simulink model "pi_8_8PSK_sim"  (Simulink 8.3)
settings: Solver=ode45  StartTime=0.0  StopTime=10  MaxStep=1e-3  RelTol=1e-3
libraries: dspobslib x2, commdigbbndpm3 x2, commchan3 x1, commsink2 x1, commutil2 x1, commrandsrc2 x1
settings Model: Creator=hlzhang  LastModifiedBy=hlzhang
settings DataIOCC: SignalLoggingName=sigsOut
settings DebuggingCC: SaveWithParameterizedLinksMsg=none  SignalResolutionControl=TryResolveAllWithWarning  SolverPrmCheckMsg=none  MultiTaskDSMMsg=warning  MultiTaskCondExecSysMsg=none  StateNameClashWarn=none
settings HardwareCC: TargetUnknown=on
settings RTWCC: IncludeERTFirstTime=on

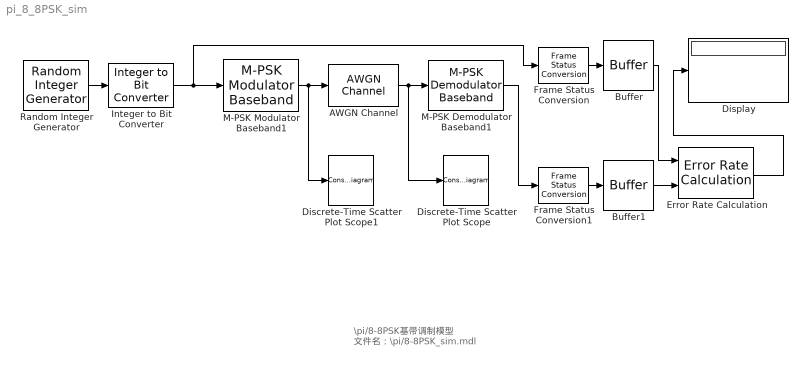
== system pi_8_8PSK_sim ==
  note: \pi/8-8PSK基带调制模型
      | 文件名：\pi/8-8PSK_sim.mdl
  AWGN Channel : commchan3/AWGN Channel  InputProcessing=Inherited (this choice will be removed - see release notes)  seed=67  noiseMode=Variance from mask  EbNodB=10  EsNodB=10  SNRdB=10  bitsPerSym=1  Ps=1  Tsym=1e-3  variance=0.02
  Buffer : Buffer  N=1
  Buffer1 : Buffer  N=1
  Discrete-Time Scatter Plot Scope : ConstellationDiagram  Tag=ScatterPlot  ScopeSpecification=DataTag1
  Discrete-Time Scatter Plot Scope1 : ConstellationDiagram  Tag=ScatterPlot  ScopeSpecification=DataTag2
  Display : Display
  Error Rate Calculation : commsink2/Error Rate Calculation  N=0  st_delay=0  cp_mode=Entire frame  subframe=[]  PMode=Port  WsName=ErrorVec  RsMode2=off  stop=off  numErr=100  maxBits=1e6
  Frame Status Conversion : dspobslib/Frame Status Conversion  growRefPort=off  outframe=Frame-based
  Frame Status Conversion1 : dspobslib/Frame Status Conversion  growRefPort=off  outframe=Frame-based
  Integer to Bit Converter : commutil2/Integer to Bit Converter  nbits=3  signedInputValues=Unsigned  bitOrder=MSB first  outDtype=Inherit via internal rule
  M-PSK Demodulator Baseband1 : commdigbbndpm3/M-PSK Demodulator Baseband  M=8  Ph=pi/8  Dec=Gray  Mapping=[0:7]  OutType=Bit  DecType=Hard decision  VarSource=Dialog  Variance=1  outDtype1=Inherit via internal rule  outDtype2=Inherit via internal rule  derotateFactorWordLen=16
  M-PSK Modulator Baseband1 : commdigbbndpm3/M-PSK Modulator Baseband  M=8  InType=Bit  Enc=Gray  Mapping=[0:7]  Ph=pi/8  outDtype=double  outWordLen=16  outUDDataType=sfix(16)  outFracLenMode=Best precision  outFracLen=15
  Random Integer Generator : commrandsrc2/Random Integer Generator  mul=8  seed=3  Ts=1e-3  frameBased=off  sampPerFrame=1  orient=off  outDataType=double
  wires:
  Random Integer Generator/1 -> Integer to Bit Converter/1
  Buffer1/1 -> Error Rate Calculation/2
  Frame Status Conversion/1 -> Buffer/1
  Frame Status Conversion1/1 -> Buffer1/1
  Integer to Bit Converter/1 -> M-PSK Modulator Baseband1/1, Frame Status Conversion/1
  M-PSK Modulator Baseband1/1 -> AWGN Channel/1, Discrete-Time Scatter Plot Scope1/1
  AWGN Channel/1 -> M-PSK Demodulator Baseband1/1, Discrete-Time Scatter Plot Scope/1
  Buffer/1 -> Error Rate Calculation/1
  M-PSK Demodulator Baseband1/1 -> Frame Status Conversion1/1
  Error Rate Calculation/1 -> Display/1
